simulink model "Práctica 1 Simulink"  (R2024b)
settings: Solver=VariableStepAuto  StartTime=0.0  StopTime=10  RelTol=1e-3
InitFcn:
  | Ip=0.0079;
  | Mc=0.7031;
  | lp=0.3302;
  | Mp=0.23;
  | Fc=0;
  | Beq=4.3;
  | g=9.81;
  | Bp=0.0024;
  | z1=0;
  | z2=0;
  | z3=1;
  | z4=0;

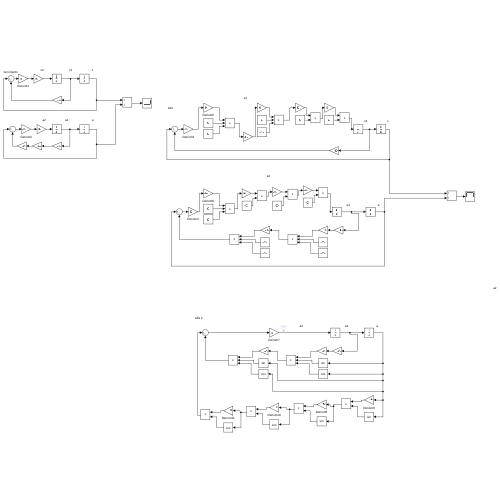
[thumbnail: Simulink's stored preview of the top-level diagram]
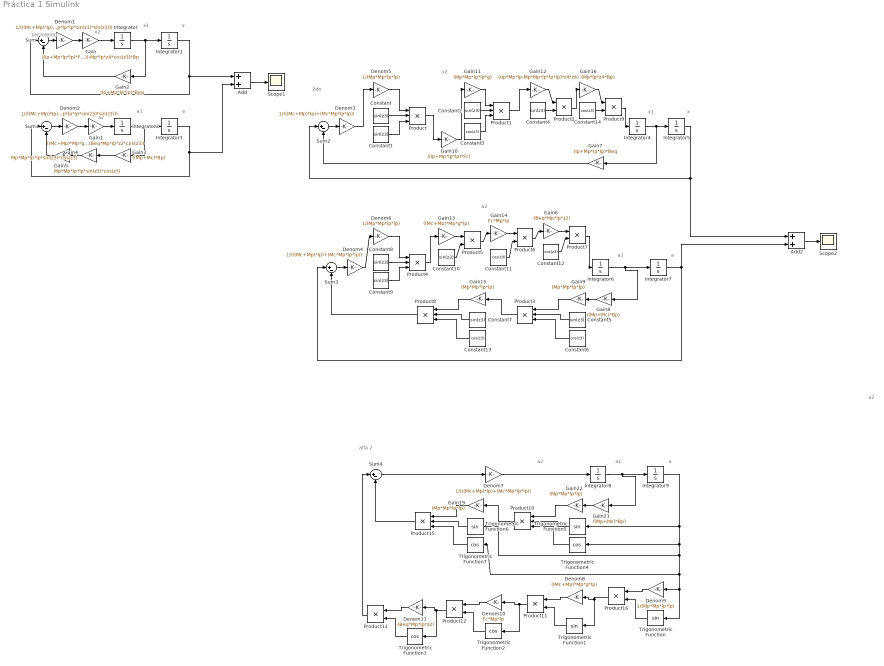
== system Práctica 1 Simulink ==
  note: alfa 2
  note: 2do
  note: 1er intento
  note: x2
  note: x1
  note: x
  note: a2
  note: a1
  note: a
  note: x2
  note: a1
  note: x
  note: x1
  note: a
  note: a2
  note: a1
  note: a2
  note: a
  note: a2
  Add : Sum
  Add2 : Sum
  Constant{,1..2,4..5,7..10} (9 alike) : Constant  Value=sin(z3)
  Constant{3,6,11..14} (6 alike) : Constant  Value=cos(z3)
  Denom1 : Gain  Gain=1/(((Mc+Mp)*Ip)+(Mc*Mp*lp*lp)+(Mp*Mp*lp*lp*sin(z3)*sin(z3)))
  Denom10 : Gain  Gain=Fc*Mp*lp
  Denom11 : Gain  Gain=-(Beq*Mp*lp*z2)
  Denom2 : Gain  Gain=1/(((Mc+Mp)*Ip)+(Mc*Mp*lp*lp)+(Mp*Mp*lp*lp*sin(z3)*sin(z3)))
  Denom3 : Gain  Gain=1/(((Mc+Mp)*Ip)+(Mc*Mp*lp*lp))
  Denom4 : Gain  Gain=1/(((Mc+Mp)*Ip)+(Mc*Mp*lp*lp))
  Denom5 : Gain  Gain=1/(Mp*Mp*lp*lp)
  Denom6 : Gain  Gain=1/(Mp*Mp*lp*lp)
  Denom7 : Gain  Gain=1/(((Mc+Mp)*Ip)+(Mc*Mp*lp*lp))
  Denom8 : Gain  Gain=((Mc+Mp)*Mp*g*lp)
  Denom9 : Gain  Gain=1/(Mp*Mp*lp*lp)
  Gain : Gain  Gain=((Ip+Mp*lp*lp)*Fc)+(Mp*Mp*lp*lp*g*cos(z3)*sin(z3))-((Ip*Mp*lp-Mp*Mp*lp*lp*lp)*z4*z4*sin(z3))-Mp*lp*z4*cos(z3)*Bp
  Gain1 : Gain  Gain=((Mc+Mp)*Mp*g*lp*sin(z3))+(Fc*Mp*lp*cos(z3))-(Beq*Mp*lp*z2*cos(z3))
  Gain10 : Gain  Gain=((Ip+Mp*lp*lp)*Fc)
  Gain11 : Gain  Gain=(Mp*Mp*lp*lp*g)
  Gain12 : Gain  Gain=-((Ip*Mp*lp-Mp*Mp*lp*lp*lp)*z4*z4)
  Gain13 : Gain  Gain=((Mc+Mp)*Mp*g*lp)
  Gain14 : Gain  Gain=Fc*Mp*lp
  Gain{9,15,19,22} (4 alike) : Gain  Gain=(Mp*Mp*lp*lp)
  Gain16 : Gain  Gain=-(Mp*lp*z4*Bp)
  Gain2 : Gain  Gain=(Ip+Mp*lp*lp)*Beq
  Gain21 : Gain  Gain=((Mp+Mc)*Bp)
  Gain3 : Gain  Gain=((Mp+Mc)*Bp)
  Gain4 : Gain  Gain=Mp*Mp*lp*lp*sin(z3)*cos(z3)
  Gain5 : Gain  Gain=Mp*Mp*lp*lp*sin(z3)*cos(z3)
  Gain6 : Gain  Gain=-(Beq*Mp*lp*z2)
  Gain7 : Gain  Gain=(Ip+Mp*lp*lp)*Beq
  Gain8 : Gain  Gain=((Mp+Mc)*Bp)
  Integrator{,1..2,4..6,8} (7 alike) : Integrator
  Integrator3 : Integrator  InitialCondition=1
  Integrator7 : Integrator  InitialCondition=1
  Integrator9 : Integrator  InitialCondition=1
  Product{,1,3..4,8,10,15} (7 alike) : Product  Inputs=3
  Product{2,5..7,9,11..13,16} (9 alike) : Product
  Scope1 : Scope
  Scope2 : Scope
  Sum{,1..4} (5 alike) : Sum  Inputs=|+-
  Trigonometric Function{,1,5..6} (4 alike) : Trigonometry
  Trigonometric Function{2..4,7} (4 alike) : Trigonometry  Operator=cos
  wires:
  Gain/1 -> Integrator/1
  Integrator/1 -> Gain2/1, Integrator1/1
  Gain2/1 -> Sum/2
  Integrator1/1 -> Sum/1, Add/1
  Sum/1 -> Denom1/1
  Denom1/1 -> Gain/1
  Sum1/1 -> Denom2/1
  Denom2/1 -> Gain1/1
  Gain1/1 -> Integrator2/1
  Integrator2/1 -> Gain3/1, Integrator3/1
  Gain3/1 -> Gain4/1
  Gain4/1 -> Gain5/1
  Integrator3/1 -> Add/2, Sum1/1
  Add/1 -> Scope1/1
  Integrator5/1 -> Add2/1, Sum2/1
  Gain7/1 -> Sum2/2
  Integrator4/1 -> Gain7/1, Integrator5/1
  Integrator7/1 -> Sum3/1, Add2/2
  Gain8/1 -> Gain9/1
  Sum2/1 -> Denom3/1
  Sum3/1 -> Denom4/1
  Integrator6/1 -> Gain8/1, Integrator7/1
  Denom5/1 -> Product/1
  Constant/1 -> Product/2
  Denom3/1 -> Denom5/1
  Product/1 -> Gain10/1
  Constant1/1 -> Product/3
  Gain10/1 -> Gain11/1
  Constant2/1 -> Product1/2
  Constant3/1 -> Product1/3
  Gain11/1 -> Product1/1
  Product1/1 -> Gain12/1
  Constant4/1 -> Product2/2
  Gain12/1 -> Product2/1
  Gain5/1 -> Sum1/2
  Gain9/1 -> Product3/1
  Constant5/1 -> Product3/2
  Constant6/1 -> Product3/3
  Constant8/1 -> Product4/2
  Denom6/1 -> Product4/1
  Denom4/1 -> Denom6/1
  Constant9/1 -> Product4/3
  Product4/1 -> Gain13/1
  Gain13/1 -> Product5/1
  Constant10/1 -> Product5/2
  Product5/1 -> Gain14/1
  Gain14/1 -> Product6/1
  Constant11/1 -> Product6/2
  Product6/1 -> Gain6/1
  Gain6/1 -> Product7/1
  Constant12/1 -> Product7/2
  Product7/1 -> Integrator6/1
  Gain15/1 -> Product8/1
  Constant13/1 -> Product8/3
  Constant7/1 -> Product8/2
  Product3/1 -> Gain15/1
  Product8/1 -> Sum3/2
  Add2/1 -> Scope2/1
  Constant14/1 -> Product9/2
  Gain16/1 -> Product9/1
  Product2/1 -> Gain16/1
  Product9/1 -> Integrator4/1
  Product10/1 -> Gain19/1
  Trigonometric Function5/1 -> Product10/2
  Product15/1 -> Sum4/2
  Gain19/1 -> Product15/1
  Trigonometric Function7/1 -> Product15/3
  Integrator9/1 -> Trigonometric Function5/1, Trigonometric Function4/1, Trigonometric Function6/1, Trigonometric Function7/1, Trigonometric Function/1, Denom9/1
  Gain22/1 -> Product10/1
  Denom7/1 -> Integrator8/1
  Trigonometric Function6/1 -> Product15/2
  Trigonometric Function4/1 -> Product10/3
  Sum4/1 -> Denom7/1
  Integrator8/1 -> Gain21/1, Integrator9/1
  Gain21/1 -> Gain22/1
  Trigonometric Function/1 -> Product16/2
  Denom9/1 -> Product16/1
  Trigonometric Function1/1 -> Product11/2
  Denom8/1 -> Product11/1
  Product16/1 -> Trigonometric Function1/1, Denom8/1
  Trigonometric Function2/1 -> Product12/2
  Denom10/1 -> Product12/1
  Product11/1 -> Trigonometric Function2/1, Denom10/1
  Trigonometric Function3/1 -> Product13/2
  Denom11/1 -> Product13/1
  Product12/1 -> Trigonometric Function3/1, Denom11/1
  Product13/1 -> Sum4/1
